simulink model "Block_diagram"  (R2025a)
settings: Solver=VariableStepAuto  StartTime=0.0  StopTime=10.0  RelTol=1e-3
settings Model: Creator=ADEEB  LastModifiedBy=ADEEB

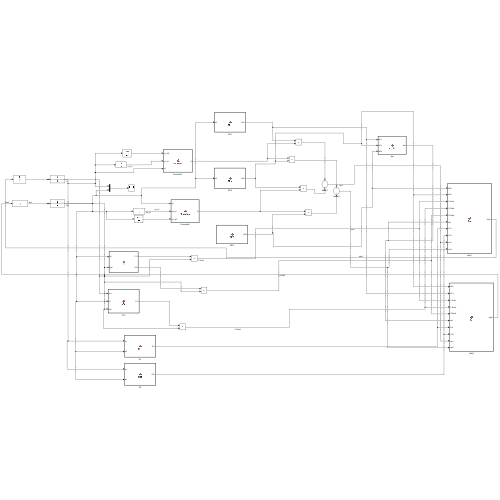
[thumbnail: Simulink's stored preview of the top-level diagram]
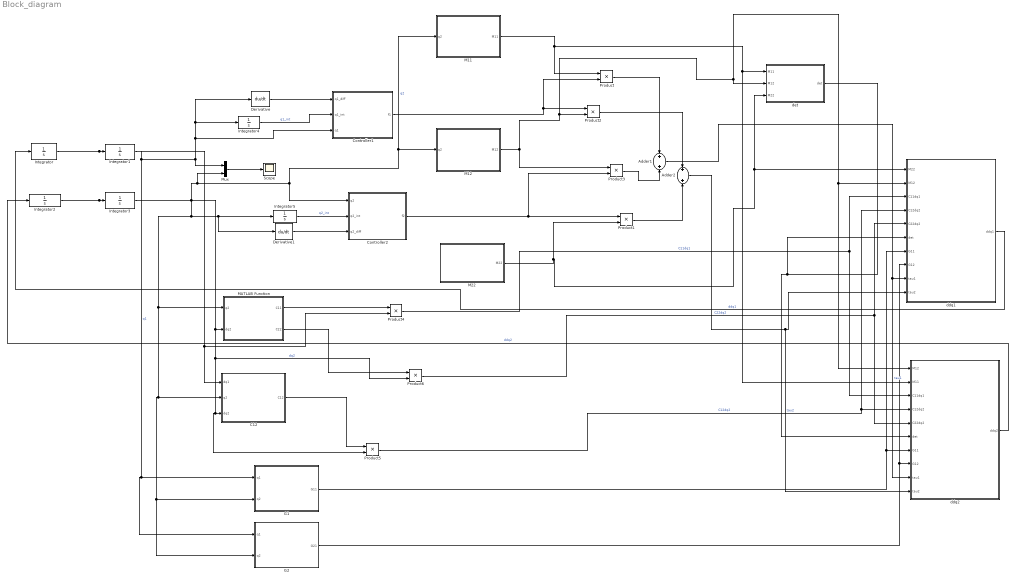
== system Block_diagram ==
  Adder1 : Sum  Inputs=+|+
  Adder2 : Sum  Inputs=+|+
  C12 : MATLAB Function  TreatAsAtomicUnit=on
  Controller1 : MATLAB Function  TreatAsAtomicUnit=on
  Controller2 : MATLAB Function  TreatAsAtomicUnit=on
  Derivative : Derivative
  Derivative1 : Derivative
  G1 : MATLAB Function  TreatAsAtomicUnit=on
  G2 : MATLAB Function  TreatAsAtomicUnit=on
  Integrator{,2,4..5} (4 alike) : Integrator
  Integrator1 : Integrator  InitialCondition=0.2
  Integrator3 : Integrator  InitialCondition=0.15
  M11 : MATLAB Function  TreatAsAtomicUnit=on
  M12 : MATLAB Function  TreatAsAtomicUnit=on
  M22 : MATLAB Function  TreatAsAtomicUnit=on
  MATLAB Function : MATLAB Function  TreatAsAtomicUnit=on
  Mux : Mux  Inputs=2
  Product{,1..6} (7 alike) : Product
  Scope : Scope
      settings: ActiveDisplayYMinimum=-1.1287933506800003  ActiveDisplayYMaximum=1.2219369622188732
  ddq1 : MATLAB Function  TreatAsAtomicUnit=on
  ddq2 : MATLAB Function  TreatAsAtomicUnit=on
  det : MATLAB Function  TreatAsAtomicUnit=on
  wires:
  M22/1(M22) -> det/3(M22), ddq1/1(M22), Product1/2
  Product3/1 -> Adder1/2
  Product/1 -> Adder1/1
  ddq2/1(ddq2) -> Integrator2/1  "ddq2"
  Derivative/1 -> Controller1/1(q1_diff)
  Product5/1 -> ddq1/4(C12dq2), ddq2/4(C12dq2)  "C12dq2"
  Product2/1 -> Adder2/1
  M12/1(M12) -> ddq2/1(M12), ddq1/2(M12), det/2(M12), Product2/2, Product3/1
  Derivative1/1 -> Controller2/3(q2_diff)
  MATLAB Function/1(C11) -> Product4/1
  Integrator/1 -> Integrator1/1, C12/1(dq1), Product4/2
  Adder1/1 -> ddq2/9(tau1), ddq1/9(tau1)  "tau1"
  MATLAB Function/2(C22) -> Product6/1
  Product6/1 -> ddq1/5(C22dq2), ddq2/5(C22dq2)  "C22dq2"
  Product1/1 -> Adder2/2
  Integrator2/1 -> Product5/2, C12/3(dq2), Product6/2, MATLAB Function/2(dq2), Integrator3/1  "dq2"
  det/1(det) -> ddq2/6(det), ddq1/6(det)
  Integrator4/1 -> Controller1/2(q1_int)  "q1_int"
  M11/1(M11) -> Product/1, ddq2/2(M11), det/1(M11)
  G2/1(G21) -> ddq1/8(G12), ddq2/8(G12)
  Controller2/1(f2) -> Product3/2, Product1/1
  C12/1(C12) -> Product5/1
  Controller1/1(f1) -> Product2/1, Product/2
  Integrator1/1 -> G2/1(q1), G1/1(q1), Derivative/1, Integrator4/1, Controller1/3(q1), Mux/1  "q1"
  Integrator5/1 -> Controller2/2(q2_int)  "q2_int"
  Product4/1 -> ddq2/3(C11dq1), ddq1/3(C11dq1)  "C11dq1"
  Adder2/1 -> ddq1/10(tau2), ddq2/10(tau2)  "tau2"
  ddq1/1(ddq1) -> Integrator/1  "ddq1"
  Integrator3/1 -> Derivative1/1, Integrator5/1, G2/2(q2), G1/2(q2), C12/2(q2), MATLAB Function/1(q2), Mux/2, Controller2/1(q2), M11/1(q2), M12/1(q2)  "q2"
  G1/1(G11) -> ddq1/7(G11), ddq2/7(G11)
  Mux/1 -> Scope/1

== matlab function Block_diagram/ddq2 ==
  data: M12 input; ddq2 output; M11 input; C11dq1 input; C12dq2 input; C22dq2 input; det input; G11 input; G12 input; tau1 input; tau2 input
function ddq2 = fcn(M12,M11,C11dq1,C12dq2,C22dq2,det,G11,G12,tau1,tau2)
Z1 = (M12*(C11dq1+C12dq2)- M11*C22dq2)./det;
Z2 = (M12*G11 - M11*G12)./det;
Z3 = (-M12*tau1 + M11*tau2)./det;
ddq2 = Z1 + Z2 + Z3 ;
end

== matlab function Block_diagram/M12 ==
  data: q2 input; M12 output
function M12 = M12(q2)
m_2 = 3;
l_1 = 0.25;
l_2 = 0.15;
M12 = m_2*l_2*(l_2 + l_1*cos(q2));
end

== matlab function Block_diagram/M11 ==
  data: q2 input; M11 output
function M11 = M11(q2)
m_1 = 5;
m_2 = 3;
l_1 = 0.25;
l_2 = 0.15;
M11 = (m_1 + m_2)*l_1^2 + m_2*l_2*(l_2 + 2*l_1*cos(q2));
end

== matlab function Block_diagram/M22 ==
  data: M22 output
function M22 = M22()
m_2 = 3;
l_2 = 0.15;
M22 = m_2*l_2^2;
end

== matlab function Block_diagram/MATLAB Function ==
  data: q2 input; C11 output; dq2 input; C22 output
function [C11,C22] = C11(q2,dq2)
m_2 = 3;
l_1 = 0.25;
l_2 = 0.15;
C11 = -(m_2*l_1*l_2*sin(q2)*dq2);
C22 = -C11;
end

== matlab function Block_diagram/C12 ==
  data: dq1 input; q2 input; C12 output; dq2 input
function C12 = C12(dq1,q2, dq2)
m_2 = 3;
l_1 = 0.25;
l_2 = 0.15;
C12 = -m_2*l_1*l_2*sin(q2)*(dq1+dq2);
end

== matlab function Block_diagram/G1 ==
  data: q1 input; q2 input; G11 output
function G11 = G11(q1, q2)
m_1 = 5;
m_2 = 3;
l_1 = 0.25;
l_2 = 0.15;
g = 9.81;
G11 = m_1*l_1*g*cos(q1) + m_2*g*(l_2*cos(q1+q2) + l_1*cos(q1));
end

== matlab function Block_diagram/G2 ==
  data: q1 input; q2 input; G21 output
function G21 = G21(q1, q2)
m_2 = 3;
l_2 = 0.15;
g = 9.81;
G21 = m_2*g*l_2*cos(q1+q2);
end

== matlab function Block_diagram/Controller1 ==
  data: q1_diff input; q1_int input; q1 input; f1 output
function f1 = Controller1(q1_diff, q1_int, q1)
Kp=200;
Ki=0;
Kd=40;
q_desired=0;
f1 = Kp * (q_desired - q1) - Kd * q1_diff - Ki * q1_int;
end

== matlab function Block_diagram/Controller2 ==
  data: q2 input; f2 output; q2_int input; q2_diff input
function f2 = Controller2(q2, q2_int, q2_diff)
Kp=20;
Ki=0;
Kd=6;
q_desired=0;
f2 = Kp * (q_desired - q2) - Kd * q2_diff - Ki * q2_int;
end

== matlab function Block_diagram/det ==
  data: M11 input; det output; M12 input; M22 input
function det = det_M(M11,M12,M22)
det = M11*M22 - M12^2;
end

== matlab function Block_diagram/ddq1 ==
  data: M22 input; ddq1 output; M12 input; C11dq1 input; C12dq2 input; C22dq2 input; det input; G11 input; G12 input; tau1 input; tau2 input
function ddq1 = fcn(M22,M12,C11dq1,C12dq2,C22dq2,det,G11,G12,tau1,tau2)
Z1 = (-M22*(C11dq1+C12dq2)+M12*C22dq2)./det;
Z2 = (-M22*G11+M12*G12)./det;
Z3 = (M22*tau1 - M12*tau2)./det;
ddq1 = Z1 + Z2 + Z3 ;
end
